simulink model "sampleModel1543_sub_sub_sub"  (R2023a)
settings: Solver=VariableStepAuto  StartTime=0.0  StopTime=10.0  RelTol=1e-3
libraries: hdlsllib x5, simulink x3
settings Model: Creator=user1  LastModifiedBy=user1
settings OptimizationCC: BlockReduction=off  ConditionallyExecuteInputs=off

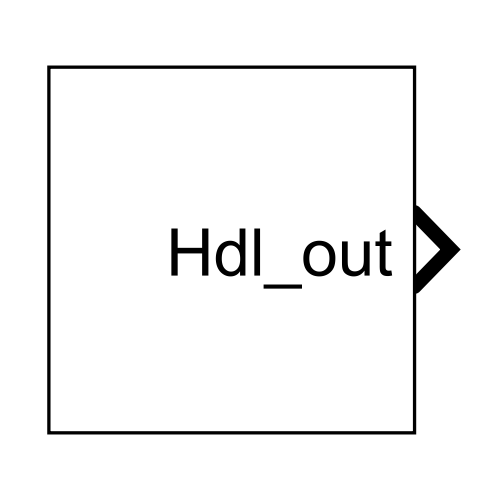
[thumbnail: Simulink's stored preview of the top-level diagram]
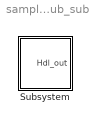
== system sampleModel1543_sub_sub_sub ==
  Subsystem : Subsystem

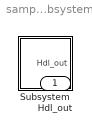
== system sampleModel1543_sub_sub_sub/Subsystem ==
  Subsystem : Subsystem
  Hdl_out : Outport  OutDataTypeStr=uint8

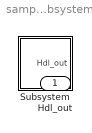
== system sampleModel1543_sub_sub_sub/Subsystem/Subsystem ==
  Subsystem : Subsystem
  Hdl_out : Outport  OutDataTypeStr=uint8

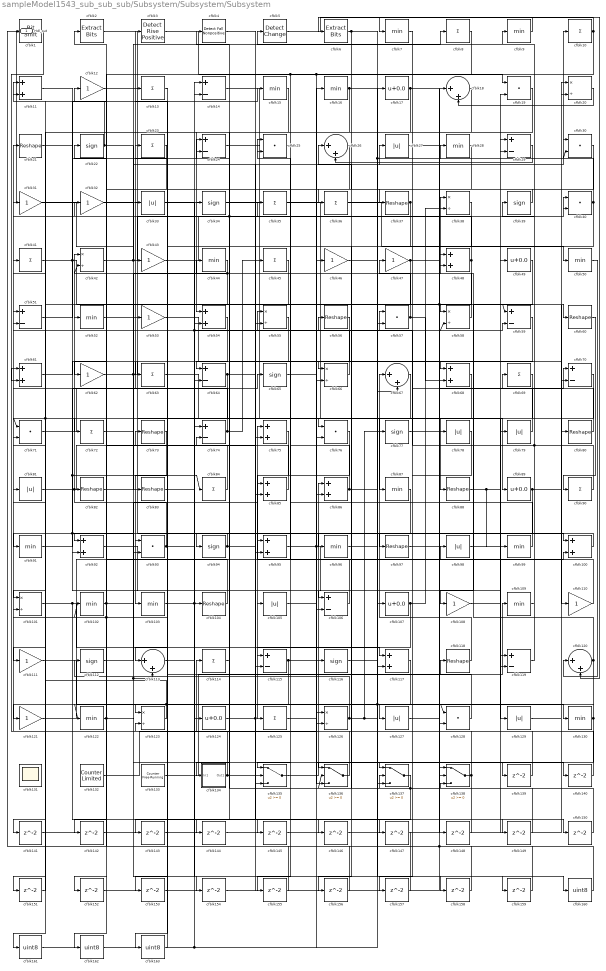
== system sampleModel1543_sub_sub_sub/Subsystem/Subsystem/Subsystem ==
  cfblk1 : hdlsllib/Logic and Bit Operations/Bit Shift  mode=Shift Left Logical  N=0
  cfblk{8,10,13,23,35..36,41,45,63,69,72,84,90,114,125} (15 alike) : Sum  Inputs=+  OutDataTypeStr=uint8
  cfblk{11,48,54,61,68,75,85..86,92,95,100,117} (12 alike) : Sum  OutDataTypeStr=uint8
  cfblk{20,38,42,55,58,66,101,123,126} (9 alike) : Product  Inputs=*/  OutDataTypeStr=uint8  RndMeth=Zero  SaturateOnIntegerOverflow=on
  cfblk{7,9,15..16,28,44,50,52,87,91,96,99,102..103,109,122,130} (17 alike) : MinMax  OutDataTypeStr=uint8
  cfblk{21,37,56,60,73,80,82..83,88,97,104,118} (12 alike) : Reshape
  cfblk{27,33,78..79,81,98,105,127,129} (9 alike) : Abs  OutDataTypeStr=uint8  SaturateOnIntegerOverflow=off
  cfblk{14,24,29,51,59,64,70,74,106,115,119} (11 alike) : Sum  Inputs=+-  OutDataTypeStr=uint8
  cfblk{17,49,89,107,124} (5 alike) : Bias  Bias=0.0  SaturateOnIntegerOverflow=off
  cfblk{12,31..32,43,46..47,53,62,108,110..111,121} (12 alike) : Gain  OutDataTypeStr=uint8
  cfblk{22,34,39,65,77,94,112,116} (8 alike) : Signum
  cfblk{18,26,67,113,120} (5 alike) : Sum  Inputs=|++  OutDataTypeStr=uint8
  cfblk{19,25,30,40,57,71,76,93,128} (9 alike) : DotProduct  OutDataTypeStr=uint8
  cfblk131 : Scope
      settings: Floating=on
  cfblk132 : hdlsllib/Sources/Counter Limited  uplimit=7  tsamp=-1
  cfblk133 : hdlsllib/Sources/Counter Free-Running  NumBits=16  tsamp=-1
  cfblk134 : Subsystem
      settings: LibrarySourceBlock=|
      | hdlsllib/Ports &
      | Subsystems/Subsystem
  cfblk{135..138} (4 alike) : Switch  OutDataTypeStr=uint8  SaturateOnIntegerOverflow=off  InputSameDT=off
  cfblk{139..159} (21 alike) : Delay  SampleTime=1
  cfblk{160..163} (4 alike) : DataTypeConversion  OutDataTypeStr=uint8  SaturateOnIntegerOverflow=off  RndMeth=Floor
  cfblk2 : simulink/Logic and Bit Operations/Extract Bits  bitsToExtract=Upper half  numBits=8  bitIdxRange=[0 7]  outScalingMode=Preserve fixed-point scaling
      settings: LibrarySourceBlock=|
      | hdlsllib/Logic and Bit
      | Operations/Extract Bits
  cfblk3 : hdlsllib/Logic and Bit Operations/Detect Rise Positive  vinit=0  OutDataTypeStr=uint8
  cfblk4 : hdlsllib/Logic and Bit Operations/Detect Fall Nonpositive  vinit=0  OutDataTypeStr=uint8
  cfblk5 : simulink/Logic and Bit Operations/Detect Change  vinit=0  OutDataTypeStr=uint8
      settings: LibrarySourceBlock=|
      | hdlsllib/Logic and Bit
      | Operations/Detect
      | Change
  cfblk6 : simulink/Logic and Bit Operations/Extract Bits  bitsToExtract=Upper half  numBits=8  bitIdxRange=[0 7]  outScalingMode=Preserve fixed-point scaling
      settings: LibrarySourceBlock=|
      | hdlsllib/Logic and Bit
      | Operations/Extract Bits
  Hdl_out : Outport  OutDataTypeStr=uint8
  wires:
  cfblk74/1 -> cfblk45/1, cfblk21/1
  cfblk118/1 -> cfblk67/1
  cfblk40/1 -> cfblk156/1, cfblk10/1
  cfblk120/1 -> cfblk144/1, cfblk48/2
  cfblk80/1 -> cfblk5/1
  cfblk2/1 -> cfblk97/1
  cfblk42/1 -> cfblk30/1, cfblk40/1
  cfblk103/1 -> cfblk159/1, cfblk58/2, cfblk48/1
  cfblk14/1 -> cfblk76/1
  cfblk138/1 -> cfblk137/2, cfblk51/1
  cfblk60/1 -> cfblk90/1
  cfblk81/1 -> cfblk55/2, cfblk42/1
  cfblk26/1 -> cfblk62/1
  cfblk73/1 -> cfblk103/1
  cfblk35/1 -> cfblk89/1
  cfblk119/1 -> cfblk69/1
  cfblk12/1 -> cfblk88/1
  cfblk31/1 -> cfblk83/1
  cfblk50/1 -> cfblk120/1
  cfblk48/1 -> cfblk145/1, cfblk4/1, cfblk11/1
  cfblk122/1 -> cfblk154/1, cfblk52/1
  cfblk134/1(Out1) -> cfblk136/1, cfblk114/1
  cfblk34/1 -> cfblk60/1
  cfblk100/1 -> cfblk92/1
  cfblk11/1 -> cfblk92/2
  cfblk18/1 -> cfblk54/1
  cfblk75/1 -> cfblk125/1
  cfblk3/1 -> cfblk19/1
  cfblk71/1 -> cfblk3/1
  cfblk8/1 -> cfblk72/1
  cfblk121/1 -> cfblk98/1
  cfblk93/1 -> cfblk100/1, cfblk2/1
  cfblk46/1 -> cfblk160/1
  cfblk54/1 -> cfblk64/1
  cfblk98/1 -> cfblk79/1
  cfblk86/1 -> cfblk25/2, cfblk30/2, cfblk17/1
  cfblk110/1 -> cfblk75/1
  cfblk33/1 -> cfblk104/1
  cfblk45/1 -> cfblk101/1
  cfblk136/1 -> cfblk33/1
  cfblk70/1 -> cfblk75/2
  cfblk111/1 -> cfblk127/1
  cfblk99/1 -> cfblk25/1
  cfblk114/1 -> cfblk74/2
  cfblk24/1 -> cfblk129/1
  cfblk5/1 -> cfblk120/2
  cfblk43/1 -> cfblk35/1
  cfblk20/1 -> cfblk18/2
  cfblk85/1 -> cfblk13/1
  cfblk130/1 -> cfblk136/3, cfblk123/1
  cfblk64/1 -> cfblk140/1, cfblk141/1, cfblk71/1
  cfblk127/1 -> cfblk78/1
  cfblk68/1 -> cfblk87/1
  cfblk135/1 -> cfblk86/1
  cfblk36/1 -> cfblk50/1
  cfblk32/1 -> cfblk8/1
  cfblk123/1 -> cfblk81/1, cfblk122/1
  cfblk62/1 -> cfblk68/1, cfblk66/1
  cfblk53/1 -> cfblk110/1
  cfblk113/1 -> cfblk117/1
  cfblk16/1 -> cfblk58/1, cfblk113/1
  cfblk58/1 -> cfblk38/1
  cfblk133/1 -> cfblk109/1
  cfblk61/1 -> cfblk63/1
  cfblk1/1 -> cfblk61/2
  cfblk17/1 -> cfblk111/1, cfblk59/1, cfblk130/1
  cfblk77/1 -> cfblk40/2
  cfblk76/1 -> cfblk105/1
  cfblk22/1 -> cfblk11/2, cfblk43/1
  cfblk51/1 -> cfblk15/1
  cfblk128/1 -> cfblk101/2
  cfblk4/1 -> cfblk106/1
  cfblk115/1 -> cfblk151/1, cfblk116/1
  cfblk108/1 -> cfblk29/2
  cfblk29/1 -> cfblk26/2
  cfblk137/1 -> cfblk143/1, cfblk136/2
  cfblk79/1 -> cfblk56/1
  cfblk25/1 -> cfblk95/1
  cfblk92/1 -> cfblk117/2
  cfblk7/1 -> cfblk37/1
  cfblk59/1 -> cfblk115/1
  cfblk44/1 -> cfblk42/2, cfblk121/1
  cfblk66/1 -> cfblk41/1
  cfblk104/1 -> cfblk12/1
  cfblk39/1 -> cfblk34/1
  cfblk15/1 -> cfblk134/1(In1)
  cfblk107/1 -> cfblk38/2, cfblk135/1
  cfblk84/1 -> cfblk22/1
  cfblk28/1 -> cfblk137/1
  cfblk63/1 -> cfblk126/1
  cfblk94/1 -> cfblk100/2, cfblk91/1
  cfblk49/1 -> cfblk108/1
  cfblk95/1 -> cfblk59/2, cfblk119/2
  cfblk124/1 -> cfblk149/1, cfblk27/1
  cfblk91/1 -> cfblk65/1
  cfblk82/1 -> cfblk44/1
  cfblk102/1 -> cfblk82/1, cfblk135/2
  cfblk129/1 -> cfblk80/1
  cfblk6/1 -> cfblk36/1, cfblk107/1
  cfblk56/1 -> cfblk94/1
  cfblk47/1 -> cfblk161/1, cfblk138/1
  cfblk125/1 -> cfblk118/1
  cfblk19/1 -> cfblk135/3
  cfblk10/1 -> cfblk7/1, cfblk76/2, cfblk155/1, cfblk115/2
  cfblk21/1 -> cfblk84/1, cfblk93/2, cfblk106/2
  cfblk101/1 -> cfblk147/1, cfblk124/1
  cfblk97/1 -> cfblk70/1
  cfblk90/1 -> cfblk9/1, cfblk57/1
  cfblk57/1 -> cfblk68/2, cfblk47/1
  cfblk132/1 -> cfblk16/1
  cfblk23/1 -> cfblk162/1
  cfblk126/1 -> cfblk112/1, cfblk77/1, cfblk28/1
  cfblk37/1 -> Hdl_out/1, cfblk93/1
  cfblk72/1 -> cfblk53/1
  cfblk41/1 -> cfblk70/2, cfblk24/1
  cfblk89/1 -> cfblk96/1, cfblk20/1
  cfblk106/1 -> cfblk55/1
  cfblk55/1 -> cfblk95/2
  cfblk65/1 -> cfblk86/2
  cfblk112/1 -> cfblk85/1
  cfblk52/1 -> cfblk137/3, cfblk113/2
  cfblk109/1 -> cfblk39/1
  cfblk88/1 -> cfblk99/1, cfblk49/1
  cfblk9/1 -> cfblk6/1
  cfblk38/1 -> cfblk126/2
  cfblk116/1 -> cfblk150/1, cfblk128/1
  cfblk96/1 -> cfblk67/2
  cfblk30/1 -> cfblk128/2
  cfblk105/1 -> cfblk139/1
  cfblk139/1 -> cfblk14/1
  cfblk140/1 -> cfblk61/1
  cfblk141/1 -> cfblk54/2
  cfblk117/1 -> cfblk142/1
  cfblk142/1 -> cfblk64/2
  cfblk143/1 -> cfblk19/2
  cfblk144/1 -> cfblk29/1
  cfblk145/1 -> cfblk20/2
  cfblk69/1 -> cfblk146/1
  cfblk146/1 -> cfblk119/1
  cfblk147/1 -> cfblk1/1
  cfblk27/1 -> cfblk148/1
  cfblk148/1 -> cfblk26/1
  cfblk149/1 -> cfblk24/2
  cfblk150/1 -> cfblk138/3
  cfblk151/1 -> cfblk51/2
  cfblk67/1 -> cfblk152/1
  cfblk152/1 -> cfblk66/2
  cfblk87/1 -> cfblk153/1
  cfblk153/1 -> cfblk18/1
  cfblk154/1 -> cfblk85/2
  cfblk155/1 -> cfblk123/2
  cfblk156/1 -> cfblk71/2
  cfblk78/1 -> cfblk157/1
  cfblk157/1 -> cfblk74/1
  cfblk83/1 -> cfblk158/1
  cfblk158/1 -> cfblk31/1
  cfblk159/1 -> cfblk73/1
  cfblk160/1 -> cfblk138/2, cfblk32/1, cfblk102/1
  cfblk161/1 -> cfblk46/1
  cfblk162/1 -> cfblk14/2, cfblk57/2
  cfblk13/1 -> cfblk163/1
  cfblk163/1 -> cfblk23/1

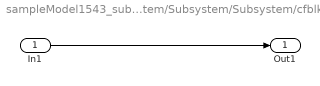
== system sampleModel1543_sub_sub_sub/Subsystem/Subsystem/Subsystem/cfblk134 ==
  In1 : Inport
  Out1 : Outport
  wires:
  In1/1 -> Out1/1
